simulink model "chap7_3sim"  (R2015a)
settings: Solver=ode45  StartTime=0.0  StopTime=10  FixedStep=0.01  RelTol=1e-3
settings Model: Creator=Masoud  LastModifiedBy=Masoud

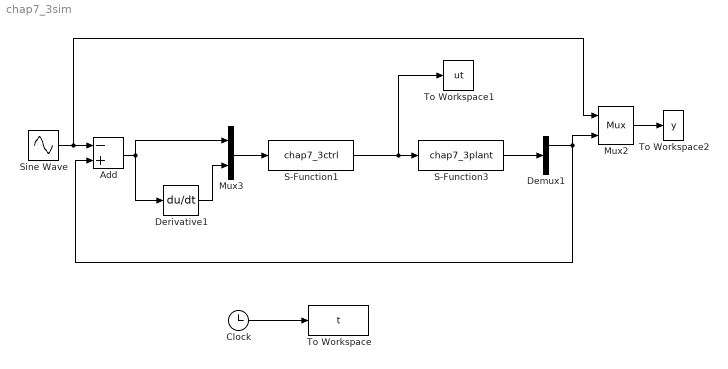
== system chap7_3sim ==
  Add : Sum  Inputs=-+
  Clock : Clock
  Demux1 : Demux  Outputs=2
  Derivative1 : Derivative
  Mux2 : Mux  Inputs=2
  Mux3 : Mux  Inputs=2
  S-Function1 : S-Function  FunctionName=chap7_3ctrl  SFunctionModules='chap7_3ctrl'
  S-Function3 : S-Function  FunctionName=chap7_3plant  SFunctionModules='chap7_3plant'
  Sine Wave : Sin  Amplitude=0.1  SampleTime=0
  To Workspace : ToWorkspace  VariableName=t  SampleTime=-1
  To Workspace1 : ToWorkspace  VariableName=ut  SampleTime=-1
  To Workspace2 : ToWorkspace  VariableName=y  SampleTime=-1
  wires:
  Clock/1 -> To Workspace/1
  Mux2/1 -> To Workspace2/1
  Mux3/1 -> S-Function1/1
  Add/1 -> Mux3/1, Derivative1/1
  Sine Wave/1 -> Mux2/1, Add/1
  Derivative1/1 -> Mux3/2
  S-Function3/1 -> Demux1/1
  Demux1/1 -> Mux2/2, Add/2
  S-Function1/1 -> To Workspace1/1, S-Function3/1
